simulink model "Ass5"  (R2024b)
settings: Solver=FixedStepAuto  StartTime=0.0  StopTime=100  FixedStep=0.2  RelTol=1e-3
libraries: simulink x1
settings Model: SnapshotBufferSize=100  SnapshotInterval=100  PacingRate=5  Creator=ArriGE66  LastModifiedBy=vise
settings ModelReferenceCC: EnableRefExpFcnMdlSchedulingChecks=on
settings RTWCC: GPUComputeCapability=3.5

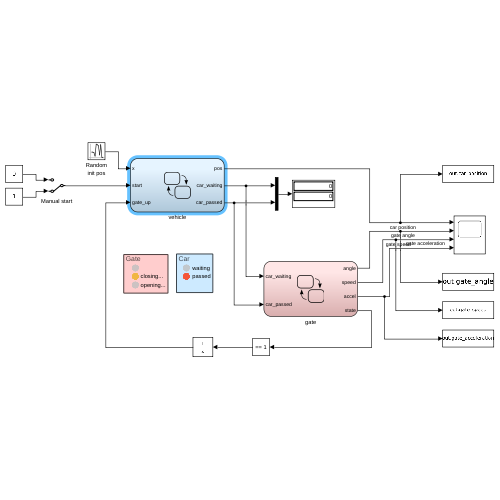
[thumbnail: Simulink's stored preview of the top-level diagram]
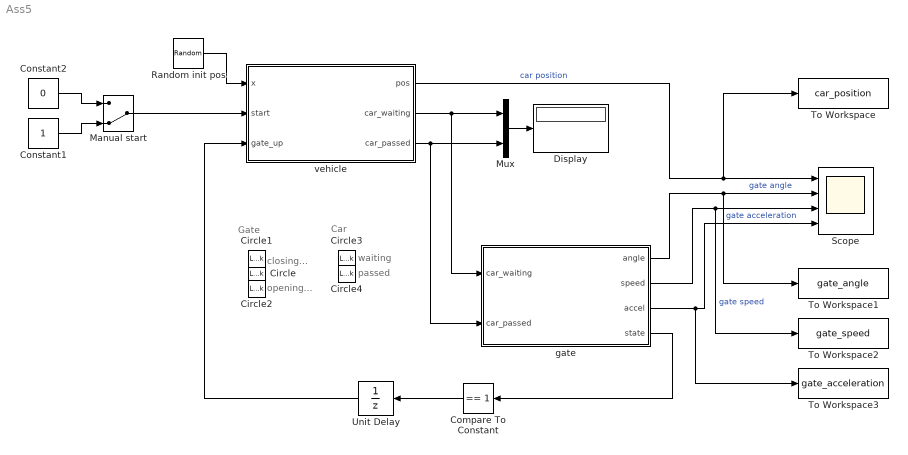
== system Ass5 ==
  note: Car
  note: waiting
  note: Gate
  note: closing...
  note: opening...
  note: passed
  Circle{,1..4} (5 alike) : LampBlock  LabelPosition=Hide  Icon=Circle
  Compare To Constant : simulink/Logic and Bit Operations/Compare To Constant  relop===  const=1  OutDataTypeStr=boolean
  Constant1 : Constant
  Constant2 : Constant  Value=0
  Display : Display
  Manual start : ManualSwitch  CurrentSetting=0
  Mux : Mux  Inputs=2
  Random init pos : RandomNumber  Mean=-15  Variance=5
  Scope : Scope  NumInputPorts=4
  To Workspace : ToWorkspace  VariableName=car_position  SampleTime=-1
      settings: Save2DSignal=2-D array (concatenate along first dimension)
  To Workspace1 : ToWorkspace  VariableName=gate_angle  SampleTime=-1
      settings: Save2DSignal=2-D array (concatenate along first dimension)
  To Workspace2 : ToWorkspace  VariableName=gate_speed  SampleTime=-1
      settings: Save2DSignal=2-D array (concatenate along first dimension)
  To Workspace3 : ToWorkspace  VariableName=gate_acceleration  SampleTime=-1
      settings: Save2DSignal=2-D array (concatenate along first dimension)
  Unit Delay : UnitDelay  SampleTime=-1  HasFrameUpgradeWarning=on
  gate : Stateflow chart  TreatAsAtomicUnit=on
  vehicle : Stateflow chart  TreatAsAtomicUnit=on
  wires:
  Random init pos/1 -> vehicle/1(x)
  Constant1/1 -> Manual start/2
  Constant2/1 -> Manual start/1
  Manual start/1 -> vehicle/2(start)
  Compare To Constant/1 -> Unit Delay/1
  vehicle/1(pos) -> To Workspace/1, Scope/1  "car position"
  Mux/1 -> Display/1
  vehicle/3(car_passed) -> gate/2(car_passed), Mux/2
  vehicle/2(car_waiting) -> gate/1(car_waiting), Mux/1
  gate/1(angle) -> To Workspace1/1, Scope/2  "gate angle"
  gate/2(speed) -> To Workspace2/1, Scope/3  "gate speed"
  gate/3(accel) -> To Workspace3/1, Scope/4  "gate acceleration"
  gate/4(state) -> Compare To Constant/1
  Unit Delay/1 -> vehicle/3(gate_up)

== stateflow chart Ass5/gate ==
  state Closed
    angle=0;
    speed=0;
    accel=0;
    state=0;
  state Rising
    state=2;
    t=elapsed(sec);
    [angle,speed,accel]=gate_moving(state,t);
  state Closing
    state=3;
    t=elapsed(sec);
    [angle,speed,accel]=gate_moving(state,t);
  state Open
    state=1;
    angle=90;
    speed=0;
    accel=0;
  (default) -> Closed
  Closing -> Closed : [angle<=0]
  Closed -> Rising : [car_waiting==1]
  Open -> Closing : [car_passed==1]
  Rising -> Open : [angle>=90]
  data: angle function_output double; speed function_output double; accel function_output double; state function_input; t function_input; car_waiting input; angle output; speed output; accel output; state output; t local; car_passed input
  function [angle,speed,accel]=gate_moving(state,t):
    | function [angle,speed,accel]=gate_moving(state,t)
    | 
    | angle=0;
    | speed=0;
    | accel=0;
    | if state == 2  % opening
    | 
    |     if t<4
    |         accel=1;
    |         angle=0.5*accel*t^2;
    |         speed=accel*t;
    |     elseif t>=4 && t<22.5
    |         speed=4;
    |         angle=8+speed*(t-4);
    |         accel=0;
    |     elseif t<=26.6
    |         accel=-1;
    |         angle=0.5*accel*(t-22.5)^2+4*(t-22.5)+82;
    |         speed=accel*(t-22.5)+4;
    |     else
    |         accel=0;
    |         angle=90;
    |         speed=0;
    |     end
    | 
    | elseif state == 3 % closing
    | 
    |     if t<4
    |         accel=-1;
    |         angle=0.5*accel*t^2+90;
    |         speed=accel*t;
    |     elseif t>=4 && t<22.5
    |         speed=-4;
    |         angle=82+speed*(t-4);
    |         accel=0;
    |     elseif t<=26.6
    |         accel=1;
    |         angle=0.5*accel*(t-22.5)^2-4*(t-22.5)+8;
    |         speed=accel*(t-22.5)-4;
    |     else
    |         accel=0;
    |         angle=0;
    |         speed=0;
    |     end
    | 
    | end
    | 
    | end

== stateflow chart Ass5/vehicle ==
  state idle
    init=x;
    pos=init;
    car_waiting=0;
    car_passed=0;
  state approaching
    pos=init+v*elapsed(sec);
  state stop
    tmp=pos;
    car_waiting=1;
    car_passed=0;
  state pass
    pos=tmp+v*elapsed(sec);
    car_waiting=0;
    ex:
    pos=tmp+v*elapsed(sec);
    tmp=pos;
  state passed
    pos=tmp+v*elapsed(sec);
    car_passed=1;
  (default) -> idle
  idle -> approaching : [start==1]
  approaching -> stop : [pos>=0]
  passed -> idle : [after(10,sec)]
  stop -> pass : [gate_up==1]
  pass -> passed : [pos>= gate_end]
  data: gate_end local =3; v local double =1; pos output; car_waiting output; car_passed output; init local; x input; start input; gate_up input; tmp local
